simulink model "Modele"  (R2013a)
settings: Solver=ode45  StartTime=0.0  StopTime=3  RelTol=1e-3
settings Model: Creator=tbesma  LastModifiedBy=dm

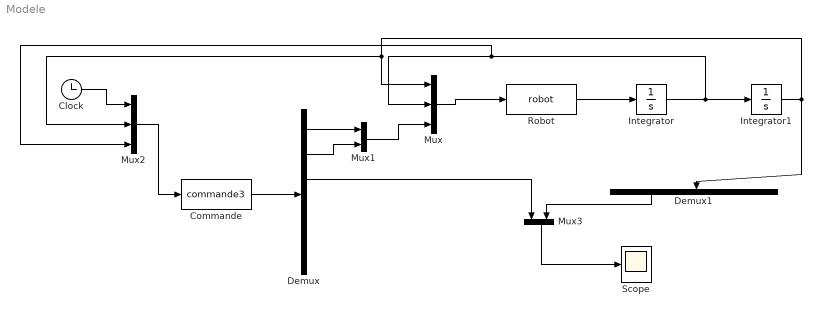
== system Modele ==
  Clock : Clock
  Commande : MATLABFcn  MATLABFcn=commande3  OutputDimensions=6
  Demux : Demux  Outputs=6
  Demux1 : Demux  Outputs=2
  Integrator : Integrator
  Integrator1 : Integrator
  Mux : Mux  Inputs=3
  Mux1 : Mux  Inputs=2
  Mux2 : Mux  Inputs=3
  Mux3 : Mux  Inputs=2
  Robot : MATLABFcn  MATLABFcn=robot  OutputDimensions=2
  Scope : Scope
      settings: ShowLegends=on  YMin=-10
  wires:
  Robot/1 -> Integrator/1
  Mux/1 -> Robot/1
  Mux2/1 -> Commande/1
  Clock/1 -> Mux2/1
  Integrator1/1 -> Demux1/1, Mux2/2, Mux/1
  Integrator/1 -> Mux2/3, Mux/2, Integrator1/1
  Commande/1 -> Demux/1
  Demux/2 -> Mux1/2
  Demux/1 -> Mux1/1
  Mux1/1 -> Mux/3
  Demux1/1 -> Mux3/2
  Demux/3 -> Mux3/1
  Mux3/1 -> Scope/1
